simulink model "微分1"  (R2018b)
settings: Solver=VariableStepAuto  StartTime=0.0  StopTime=10.0  RelTol=1e-3
settings Model: Creator=Jason  LastModifiedBy=Jason

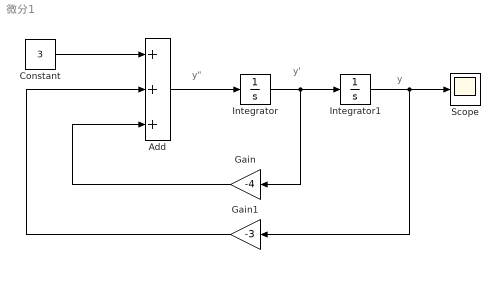
== system 微分1 ==
  note: y
  note: y'
  note: y"
  Add : Sum  Inputs=+++
  Constant : Constant  Value=3
  Gain : Gain  Gain=-4
  Gain1 : Gain  Gain=-3
  Integrator : Integrator
  Integrator1 : Integrator  InitialCondition=0.5
  Scope : Scope
  wires:
  Constant/1 -> Add/1
  Add/1 -> Integrator/1
  Integrator/1 -> Gain/1, Integrator1/1
  Gain/1 -> Add/3
  Gain1/1 -> Add/2
  Integrator1/1 -> Gain1/1, Scope/1
